simulink model "TrajectoryGenerator2DOF"  (R2023b)
settings: Solver=FixedStepDiscrete  StartTime=0.0  StopTime=1.538*1.4  FixedStep=0.002  RelTol=1e-3
undefined symbols (not defined in the file or in its folder): M_z, Smoothers, Ts
(part 1 of 3)
settings Model: Creator=simon  LastModifiedBy=simon

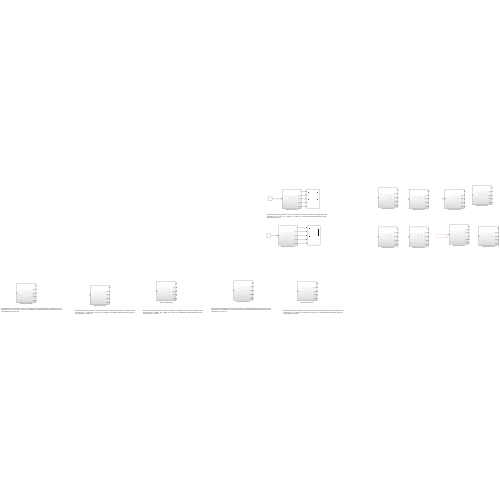
[thumbnail: Simulink's stored preview of the top-level diagram]
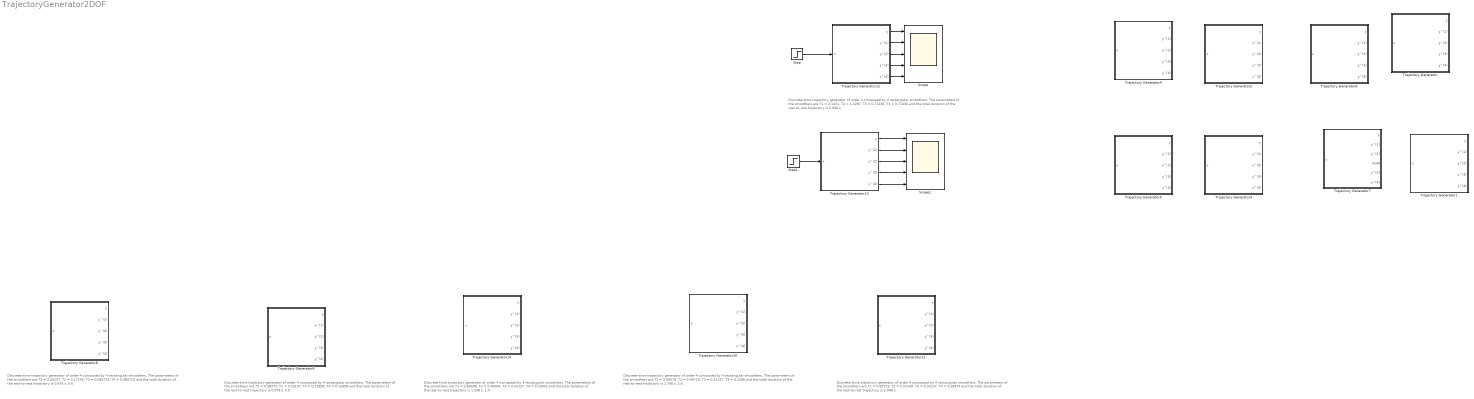
== system TrajectoryGenerator2DOF ==
  note: Discrete-time trajectory generator of order 4 composed by 4 rectangular smoothers. The parameters of the smoothers are T1 = 2.1431, T2 = 1.4287, T3 = 0.71436, T4 = 0.71436 and the total duration of the rest-to-rest trajectory is 5.006 s.
  note: Discrete-time trajectory generator of order 4 composed by 4 rectangular smoothers. The parameters of the smoothers are T1 = 0.33137, T2 = 0.17145, T3 = 0.085723, T4 = 0.085723 and the total duration of the rest-to-rest trajectory is 0.676 s. 0.6
  note: Discrete-time trajectory generator of order 4 composed by 4 rectangular smoothers. The parameters of the smoothers are T1 = 0.38575, T2 = 0.33137, T3 = 0.12858, T4 = 0.12858 and the total duration of the rest-to-rest trajectory is 0.978 s. 0.9
  note: Discrete-time trajectory generator of order 4 composed by 4 rectangular smoothers. The parameters of the smoothers are T1 = 0.68579, T2 = 0.45719, T3 = 0.33137, T4 = 0.2286 and the total duration of the rest-to-rest trajectory is 1.706 s. 1.6
  note: Discrete-time trajectory generator of order 4 composed by 4 rectangular smoothers. The parameters of the smoothers are T1 = 0.85723, T2 = 0.57149, T3 = 0.33137, T4 = 0.28574 and the total duration of the rest-to-rest trajectory is 2.048 s.
  note: Discrete-time trajectory generator of order 4 composed by 4 rectangular smoothers. The parameters of the smoothers are T1 = 0.60006, T2 = 0.40004, T3 = 0.33137, T4 = 0.20002 and the total duration of the rest-to-rest trajectory is 1.538 s. 1.4
  Scope : Scope  NumInputPorts=5
  Scope1 : Scope  NumInputPorts=5
  Step : Step  Time=0  After=0.5  SampleTime=0.002
  Step1 : Step  Time=0.4*Ts  After=-0.5  SampleTime=0.002
  Trajectory Generator : Subsystem
  Trajectory Generator1 : Subsystem
  Trajectory Generator10 : Subsystem
  Trajectory Generator11 : Subsystem
  Trajectory Generator12 : Subsystem
  Trajectory Generator13 : Subsystem
  Trajectory Generator14 : Subsystem
  Trajectory Generator2 : Subsystem
  Trajectory Generator3 : Subsystem
  Trajectory Generator4 : Subsystem
  Trajectory Generator5 : Subsystem
  Trajectory Generator6 : Subsystem
  Trajectory Generator7 : Subsystem
  Trajectory Generator8 : Subsystem
  Trajectory Generator9 : Subsystem
  wires:
  Step/1 -> Trajectory Generator12/1(x)
  Trajectory Generator12/1(y) -> Scope/1
  Trajectory Generator12/2(y^(1)) -> Scope/2
  Trajectory Generator12/3(y^(2)) -> Scope/3
  Trajectory Generator12/4(y^(3)) -> Scope/4
  Trajectory Generator12/5(y^(4)) -> Scope/5
  Step1/1 -> Trajectory Generator13/1(x)
  Trajectory Generator13/4(y^(3)) -> Scope1/4
  Trajectory Generator13/3(y^(2)) -> Scope1/3
  Trajectory Generator13/2(y^(1)) -> Scope1/2
  Trajectory Generator13/1(y) -> Scope1/1
  Trajectory Generator13/5(y^(4)) -> Scope1/5
  ? -> Trajectory Generator6/1(x)
  ? -> Trajectory Generator7/1(x)

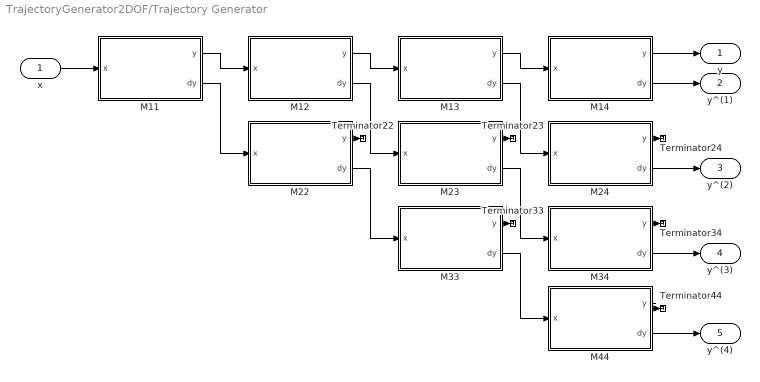
== system TrajectoryGenerator2DOF/Trajectory Generator ==
  x : Inport
  M11 : Subsystem  AncestorBlock=Smoothers/M_z  mask{N=1072, Ts=0.002, Q0=0}
      mask prompts: N "N_i"; Ts "Sampling period (Ts)"; Q0 "Initial position"
  M12 : Subsystem  AncestorBlock=Smoothers/M_z  mask{N=715, Ts=0.002, Q0=0}
      mask prompts: N "N_i"; Ts "Sampling period (Ts)"; Q0 "Initial position"
  M13 : Subsystem  AncestorBlock=Smoothers/M_z  mask{N=358, Ts=0.002, Q0=0}
      mask prompts: N "N_i"; Ts "Sampling period (Ts)"; Q0 "Initial position"
  M14 : Subsystem  AncestorBlock=Smoothers/M_z  mask{N=358, Ts=0.002, Q0=0}
      mask prompts: N "N_i"; Ts "Sampling period (Ts)"; Q0 "Initial position"
  M22 : Subsystem  AncestorBlock=Smoothers/M_z  mask{N=715, Ts=0.002, Q0=0}
      mask prompts: N "N_i"; Ts "Sampling period (Ts)"; Q0 "Initial position"
  M23 : Subsystem  AncestorBlock=Smoothers/M_z  mask{N=358, Ts=0.002, Q0=0}
      mask prompts: N "N_i"; Ts "Sampling period (Ts)"; Q0 "Initial position"
  M24 : Subsystem  AncestorBlock=Smoothers/M_z  mask{N=358, Ts=0.002, Q0=0}
      mask prompts: N "N_i"; Ts "Sampling period (Ts)"; Q0 "Initial position"
  M33 : Subsystem  AncestorBlock=Smoothers/M_z  mask{N=358, Ts=0.002, Q0=0}
      mask prompts: N "N_i"; Ts "Sampling period (Ts)"; Q0 "Initial position"
  M34 : Subsystem  AncestorBlock=Smoothers/M_z  mask{N=358, Ts=0.002, Q0=0}
      mask prompts: N "N_i"; Ts "Sampling period (Ts)"; Q0 "Initial position"
  M44 : Subsystem  AncestorBlock=Smoothers/M_z  mask{N=358, Ts=0.002, Q0=0}
      mask prompts: N "N_i"; Ts "Sampling period (Ts)"; Q0 "Initial position"
  Terminator{22..24,33..34,44} (6 alike) : Terminator
  y : Outport
  y^(1) : Outport  Port=2
  y^(2) : Outport  Port=3
  y^(3) : Outport  Port=4
  y^(4) : Outport  Port=5
  wires:
  x/1 -> M11/1(x)
  M11/1(y) -> M12/1(x)
  M12/1(y) -> M13/1(x)
  M13/1(y) -> M14/1(x)
  M11/2(dy) -> M22/1(x)
  M12/2(dy) -> M23/1(x)
  M13/2(dy) -> M24/1(x)
  M22/2(dy) -> M33/1(x)
  M23/2(dy) -> M34/1(x)
  M33/2(dy) -> M44/1(x)
  M22/1(y) -> Terminator22/1
  M23/1(y) -> Terminator23/1
  M24/1(y) -> Terminator24/1
  M33/1(y) -> Terminator33/1
  M34/1(y) -> Terminator34/1
  M44/1(y) -> Terminator44/1
  M14/1(y) -> y/1
  M14/2(dy) -> y^(1)/1
  M24/2(dy) -> y^(2)/1
  M34/2(dy) -> y^(3)/1
  M44/2(dy) -> y^(4)/1

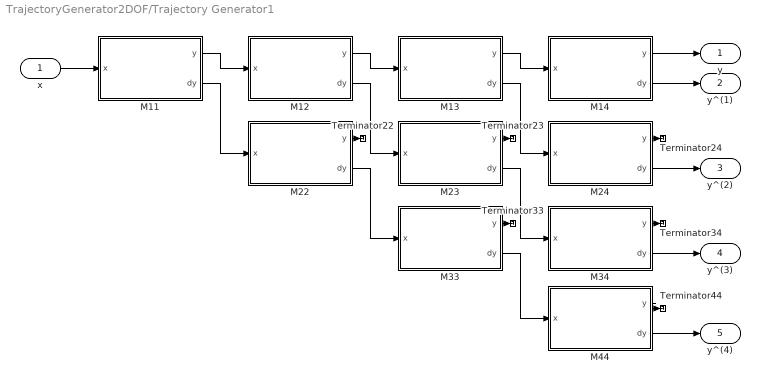
== system TrajectoryGenerator2DOF/Trajectory Generator1 ==
  x : Inport
  M11 : Subsystem  AncestorBlock=Smoothers/M_z  mask{N=1072, Ts=0.002, Q0=0}
      mask prompts: N "N_i"; Ts "Sampling period (Ts)"; Q0 "Initial position"
  M12 : Subsystem  AncestorBlock=Smoothers/M_z  mask{N=715, Ts=0.002, Q0=0}
      mask prompts: N "N_i"; Ts "Sampling period (Ts)"; Q0 "Initial position"
  M13 : Subsystem  AncestorBlock=Smoothers/M_z  mask{N=358, Ts=0.002, Q0=0}
      mask prompts: N "N_i"; Ts "Sampling period (Ts)"; Q0 "Initial position"
  M14 : Subsystem  AncestorBlock=Smoothers/M_z  mask{N=358, Ts=0.002, Q0=0}
      mask prompts: N "N_i"; Ts "Sampling period (Ts)"; Q0 "Initial position"
  M22 : Subsystem  AncestorBlock=Smoothers/M_z  mask{N=715, Ts=0.002, Q0=0}
      mask prompts: N "N_i"; Ts "Sampling period (Ts)"; Q0 "Initial position"
  M23 : Subsystem  AncestorBlock=Smoothers/M_z  mask{N=358, Ts=0.002, Q0=0}
      mask prompts: N "N_i"; Ts "Sampling period (Ts)"; Q0 "Initial position"
  M24 : Subsystem  AncestorBlock=Smoothers/M_z  mask{N=358, Ts=0.002, Q0=0}
      mask prompts: N "N_i"; Ts "Sampling period (Ts)"; Q0 "Initial position"
  M33 : Subsystem  AncestorBlock=Smoothers/M_z  mask{N=358, Ts=0.002, Q0=0}
      mask prompts: N "N_i"; Ts "Sampling period (Ts)"; Q0 "Initial position"
  M34 : Subsystem  AncestorBlock=Smoothers/M_z  mask{N=358, Ts=0.002, Q0=0}
      mask prompts: N "N_i"; Ts "Sampling period (Ts)"; Q0 "Initial position"
  M44 : Subsystem  AncestorBlock=Smoothers/M_z  mask{N=358, Ts=0.002, Q0=0}
      mask prompts: N "N_i"; Ts "Sampling period (Ts)"; Q0 "Initial position"
  Terminator{22..24,33..34,44} (6 alike) : Terminator
  y : Outport
  y^(1) : Outport  Port=2
  y^(2) : Outport  Port=3
  y^(3) : Outport  Port=4
  y^(4) : Outport  Port=5
  wires:
  M44/2(dy) -> y^(4)/1
  M34/2(dy) -> y^(3)/1
  M24/2(dy) -> y^(2)/1
  M14/2(dy) -> y^(1)/1
  M14/1(y) -> y/1
  M44/1(y) -> Terminator44/1
  M34/1(y) -> Terminator34/1
  M33/1(y) -> Terminator33/1
  M24/1(y) -> Terminator24/1
  M23/1(y) -> Terminator23/1
  M22/1(y) -> Terminator22/1
  M33/2(dy) -> M44/1(x)
  M23/2(dy) -> M34/1(x)
  M22/2(dy) -> M33/1(x)
  M13/2(dy) -> M24/1(x)
  M12/2(dy) -> M23/1(x)
  M11/2(dy) -> M22/1(x)
  M13/1(y) -> M14/1(x)
  M12/1(y) -> M13/1(x)
  M11/1(y) -> M12/1(x)
  x/1 -> M11/1(x)

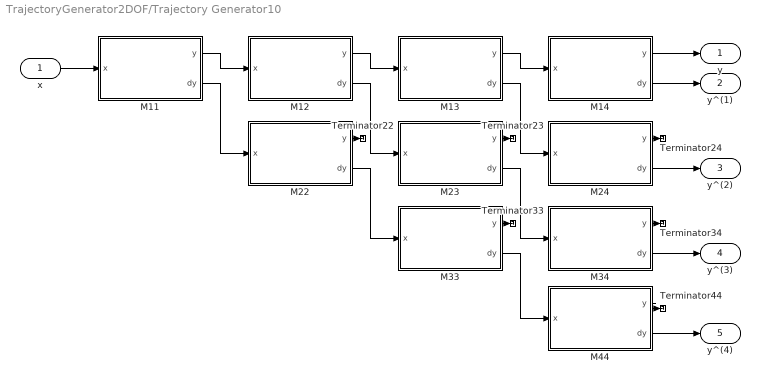
== system TrajectoryGenerator2DOF/Trajectory Generator10 ==
  x : Inport
  M11 : Subsystem  AncestorBlock=Smoothers/M_z  mask{N=343, Ts=0.002, Q0=0}
      mask prompts: N "N_i"; Ts "Sampling period (Ts)"; Q0 "Initial position"
  M12 : Subsystem  AncestorBlock=Smoothers/M_z  mask{N=229, Ts=0.002, Q0=0}
      mask prompts: N "N_i"; Ts "Sampling period (Ts)"; Q0 "Initial position"
  M13 : Subsystem  AncestorBlock=Smoothers/M_z  mask{N=166, Ts=0.002, Q0=0}
      mask prompts: N "N_i"; Ts "Sampling period (Ts)"; Q0 "Initial position"
  M14 : Subsystem  AncestorBlock=Smoothers/M_z  mask{N=115, Ts=0.002, Q0=0}
      mask prompts: N "N_i"; Ts "Sampling period (Ts)"; Q0 "Initial position"
  M22 : Subsystem  AncestorBlock=Smoothers/M_z  mask{N=229, Ts=0.002, Q0=0}
      mask prompts: N "N_i"; Ts "Sampling period (Ts)"; Q0 "Initial position"
  M23 : Subsystem  AncestorBlock=Smoothers/M_z  mask{N=166, Ts=0.002, Q0=0}
      mask prompts: N "N_i"; Ts "Sampling period (Ts)"; Q0 "Initial position"
  M24 : Subsystem  AncestorBlock=Smoothers/M_z  mask{N=115, Ts=0.002, Q0=0}
      mask prompts: N "N_i"; Ts "Sampling period (Ts)"; Q0 "Initial position"
  M33 : Subsystem  AncestorBlock=Smoothers/M_z  mask{N=166, Ts=0.002, Q0=0}
      mask prompts: N "N_i"; Ts "Sampling period (Ts)"; Q0 "Initial position"
  M34 : Subsystem  AncestorBlock=Smoothers/M_z  mask{N=115, Ts=0.002, Q0=0}
      mask prompts: N "N_i"; Ts "Sampling period (Ts)"; Q0 "Initial position"
  M44 : Subsystem  AncestorBlock=Smoothers/M_z  mask{N=115, Ts=0.002, Q0=0}
      mask prompts: N "N_i"; Ts "Sampling period (Ts)"; Q0 "Initial position"
  Terminator{22..24,33..34,44} (6 alike) : Terminator
  y : Outport
  y^(1) : Outport  Port=2
  y^(2) : Outport  Port=3
  y^(3) : Outport  Port=4
  y^(4) : Outport  Port=5
  wires:
  x/1 -> M11/1(x)
  M11/1(y) -> M12/1(x)
  M12/1(y) -> M13/1(x)
  M13/1(y) -> M14/1(x)
  M11/2(dy) -> M22/1(x)
  M12/2(dy) -> M23/1(x)
  M13/2(dy) -> M24/1(x)
  M22/2(dy) -> M33/1(x)
  M23/2(dy) -> M34/1(x)
  M33/2(dy) -> M44/1(x)
  M22/1(y) -> Terminator22/1
  M23/1(y) -> Terminator23/1
  M24/1(y) -> Terminator24/1
  M33/1(y) -> Terminator33/1
  M34/1(y) -> Terminator34/1
  M44/1(y) -> Terminator44/1
  M14/1(y) -> y/1
  M14/2(dy) -> y^(1)/1
  M24/2(dy) -> y^(2)/1
  M34/2(dy) -> y^(3)/1
  M44/2(dy) -> y^(4)/1

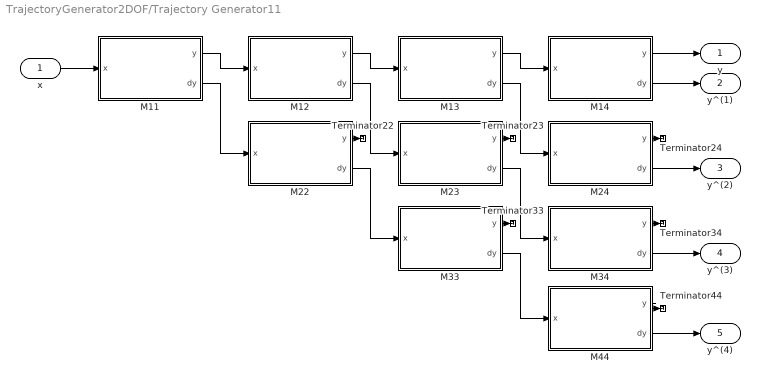
== system TrajectoryGenerator2DOF/Trajectory Generator11 ==
  x : Inport
  M11 : Subsystem  AncestorBlock=Smoothers/M_z  mask{N=429, Ts=0.002, Q0=0}
      mask prompts: N "N_i"; Ts "Sampling period (Ts)"; Q0 "Initial position"
  M12 : Subsystem  AncestorBlock=Smoothers/M_z  mask{N=286, Ts=0.002, Q0=0}
      mask prompts: N "N_i"; Ts "Sampling period (Ts)"; Q0 "Initial position"
  M13 : Subsystem  AncestorBlock=Smoothers/M_z  mask{N=166, Ts=0.002, Q0=0}
      mask prompts: N "N_i"; Ts "Sampling period (Ts)"; Q0 "Initial position"
  M14 : Subsystem  AncestorBlock=Smoothers/M_z  mask{N=143, Ts=0.002, Q0=0}
      mask prompts: N "N_i"; Ts "Sampling period (Ts)"; Q0 "Initial position"
  M22 : Subsystem  AncestorBlock=Smoothers/M_z  mask{N=286, Ts=0.002, Q0=0}
      mask prompts: N "N_i"; Ts "Sampling period (Ts)"; Q0 "Initial position"
  M23 : Subsystem  AncestorBlock=Smoothers/M_z  mask{N=166, Ts=0.002, Q0=0}
      mask prompts: N "N_i"; Ts "Sampling period (Ts)"; Q0 "Initial position"
  M24 : Subsystem  AncestorBlock=Smoothers/M_z  mask{N=143, Ts=0.002, Q0=0}
      mask prompts: N "N_i"; Ts "Sampling period (Ts)"; Q0 "Initial position"
  M33 : Subsystem  AncestorBlock=Smoothers/M_z  mask{N=166, Ts=0.002, Q0=0}
      mask prompts: N "N_i"; Ts "Sampling period (Ts)"; Q0 "Initial position"
  M34 : Subsystem  AncestorBlock=Smoothers/M_z  mask{N=143, Ts=0.002, Q0=0}
      mask prompts: N "N_i"; Ts "Sampling period (Ts)"; Q0 "Initial position"
  M44 : Subsystem  AncestorBlock=Smoothers/M_z  mask{N=143, Ts=0.002, Q0=0}
      mask prompts: N "N_i"; Ts "Sampling period (Ts)"; Q0 "Initial position"
  Terminator{22..24,33..34,44} (6 alike) : Terminator
  y : Outport
  y^(1) : Outport  Port=2
  y^(2) : Outport  Port=3
  y^(3) : Outport  Port=4
  y^(4) : Outport  Port=5
  wires:
  x/1 -> M11/1(x)
  M11/1(y) -> M12/1(x)
  M12/1(y) -> M13/1(x)
  M13/1(y) -> M14/1(x)
  M11/2(dy) -> M22/1(x)
  M12/2(dy) -> M23/1(x)
  M13/2(dy) -> M24/1(x)
  M22/2(dy) -> M33/1(x)
  M23/2(dy) -> M34/1(x)
  M33/2(dy) -> M44/1(x)
  M22/1(y) -> Terminator22/1
  M23/1(y) -> Terminator23/1
  M24/1(y) -> Terminator24/1
  M33/1(y) -> Terminator33/1
  M34/1(y) -> Terminator34/1
  M44/1(y) -> Terminator44/1
  M14/1(y) -> y/1
  M14/2(dy) -> y^(1)/1
  M24/2(dy) -> y^(2)/1
  M34/2(dy) -> y^(3)/1
  M44/2(dy) -> y^(4)/1

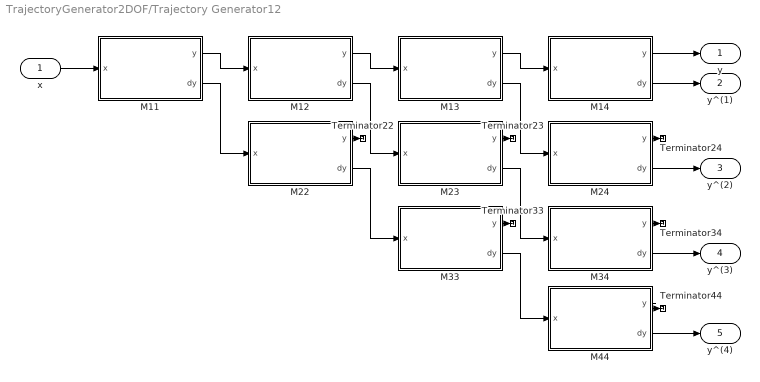
== system TrajectoryGenerator2DOF/Trajectory Generator12 ==
  x : Inport
  M11 : Subsystem  AncestorBlock=Smoothers/M_z  mask{N=301, Ts=0.002, Q0=0}
      mask prompts: N "N_i"; Ts "Sampling period (Ts)"; Q0 "Initial position"
  M12 : Subsystem  AncestorBlock=Smoothers/M_z  mask{N=201, Ts=0.002, Q0=0}
      mask prompts: N "N_i"; Ts "Sampling period (Ts)"; Q0 "Initial position"
  M13 : Subsystem  AncestorBlock=Smoothers/M_z  mask{N=166, Ts=0.002, Q0=0}
      mask prompts: N "N_i"; Ts "Sampling period (Ts)"; Q0 "Initial position"
  M14 : Subsystem  AncestorBlock=Smoothers/M_z  mask{N=101, Ts=0.002, Q0=0}
      mask prompts: N "N_i"; Ts "Sampling period (Ts)"; Q0 "Initial position"
  M22 : Subsystem  AncestorBlock=Smoothers/M_z  mask{N=201, Ts=0.002, Q0=0}
      mask prompts: N "N_i"; Ts "Sampling period (Ts)"; Q0 "Initial position"
  M23 : Subsystem  AncestorBlock=Smoothers/M_z  mask{N=166, Ts=0.002, Q0=0}
      mask prompts: N "N_i"; Ts "Sampling period (Ts)"; Q0 "Initial position"
  M24 : Subsystem  AncestorBlock=Smoothers/M_z  mask{N=101, Ts=0.002, Q0=0}
      mask prompts: N "N_i"; Ts "Sampling period (Ts)"; Q0 "Initial position"
  M33 : Subsystem  AncestorBlock=Smoothers/M_z  mask{N=166, Ts=0.002, Q0=0}
      mask prompts: N "N_i"; Ts "Sampling period (Ts)"; Q0 "Initial position"
  M34 : Subsystem  AncestorBlock=Smoothers/M_z  mask{N=101, Ts=0.002, Q0=0}
      mask prompts: N "N_i"; Ts "Sampling period (Ts)"; Q0 "Initial position"
  M44 : Subsystem  AncestorBlock=Smoothers/M_z  mask{N=101, Ts=0.002, Q0=0}
      mask prompts: N "N_i"; Ts "Sampling period (Ts)"; Q0 "Initial position"
  Terminator{22..24,33..34,44} (6 alike) : Terminator
  y : Outport
  y^(1) : Outport  Port=2
  y^(2) : Outport  Port=3
  y^(3) : Outport  Port=4
  y^(4) : Outport  Port=5
  wires:
  x/1 -> M11/1(x)
  M11/1(y) -> M12/1(x)
  M12/1(y) -> M13/1(x)
  M13/1(y) -> M14/1(x)
  M11/2(dy) -> M22/1(x)
  M12/2(dy) -> M23/1(x)
  M13/2(dy) -> M24/1(x)
  M22/2(dy) -> M33/1(x)
  M23/2(dy) -> M34/1(x)
  M33/2(dy) -> M44/1(x)
  M22/1(y) -> Terminator22/1
  M23/1(y) -> Terminator23/1
  M24/1(y) -> Terminator24/1
  M33/1(y) -> Terminator33/1
  M34/1(y) -> Terminator34/1
  M44/1(y) -> Terminator44/1
  M14/1(y) -> y/1
  M14/2(dy) -> y^(1)/1
  M24/2(dy) -> y^(2)/1
  M34/2(dy) -> y^(3)/1
  M44/2(dy) -> y^(4)/1

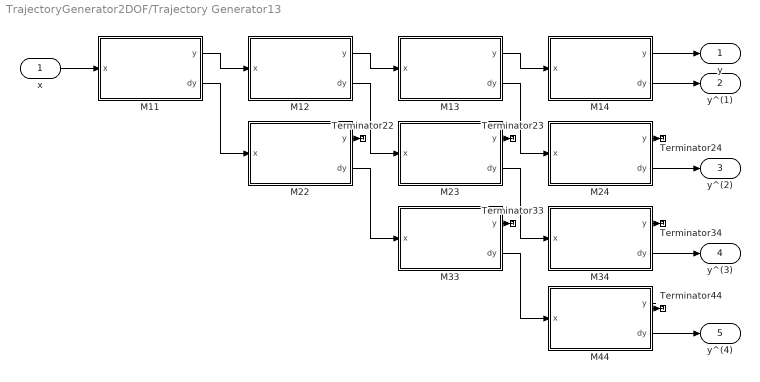
== system TrajectoryGenerator2DOF/Trajectory Generator13 ==
  x : Inport
  M11 : Subsystem  AncestorBlock=Smoothers/M_z  mask{N=301, Ts=0.002, Q0=0}
      mask prompts: N "N_i"; Ts "Sampling period (Ts)"; Q0 "Initial position"
  M12 : Subsystem  AncestorBlock=Smoothers/M_z  mask{N=201, Ts=0.002, Q0=0}
      mask prompts: N "N_i"; Ts "Sampling period (Ts)"; Q0 "Initial position"
  M13 : Subsystem  AncestorBlock=Smoothers/M_z  mask{N=166, Ts=0.002, Q0=0}
      mask prompts: N "N_i"; Ts "Sampling period (Ts)"; Q0 "Initial position"
  M14 : Subsystem  AncestorBlock=Smoothers/M_z  mask{N=101, Ts=0.002, Q0=0}
      mask prompts: N "N_i"; Ts "Sampling period (Ts)"; Q0 "Initial position"
  M22 : Subsystem  AncestorBlock=Smoothers/M_z  mask{N=201, Ts=0.002, Q0=0}
      mask prompts: N "N_i"; Ts "Sampling period (Ts)"; Q0 "Initial position"
  M23 : Subsystem  AncestorBlock=Smoothers/M_z  mask{N=166, Ts=0.002, Q0=0}
      mask prompts: N "N_i"; Ts "Sampling period (Ts)"; Q0 "Initial position"
  M24 : Subsystem  AncestorBlock=Smoothers/M_z  mask{N=101, Ts=0.002, Q0=0}
      mask prompts: N "N_i"; Ts "Sampling period (Ts)"; Q0 "Initial position"
  M33 : Subsystem  AncestorBlock=Smoothers/M_z  mask{N=166, Ts=0.002, Q0=0}
      mask prompts: N "N_i"; Ts "Sampling period (Ts)"; Q0 "Initial position"
  M34 : Subsystem  AncestorBlock=Smoothers/M_z  mask{N=101, Ts=0.002, Q0=0}
      mask prompts: N "N_i"; Ts "Sampling period (Ts)"; Q0 "Initial position"
  M44 : Subsystem  AncestorBlock=Smoothers/M_z  mask{N=101, Ts=0.002, Q0=0}
      mask prompts: N "N_i"; Ts "Sampling period (Ts)"; Q0 "Initial position"
  Terminator{22..24,33..34,44} (6 alike) : Terminator
  y : Outport
  y^(1) : Outport  Port=2
  y^(2) : Outport  Port=3
  y^(3) : Outport  Port=4
  y^(4) : Outport  Port=5
  wires:
  x/1 -> M11/1(x)
  M11/1(y) -> M12/1(x)
  M12/1(y) -> M13/1(x)
  M13/1(y) -> M14/1(x)
  M11/2(dy) -> M22/1(x)
  M12/2(dy) -> M23/1(x)
  M13/2(dy) -> M24/1(x)
  M22/2(dy) -> M33/1(x)
  M23/2(dy) -> M34/1(x)
  M33/2(dy) -> M44/1(x)
  M22/1(y) -> Terminator22/1
  M23/1(y) -> Terminator23/1
  M24/1(y) -> Terminator24/1
  M33/1(y) -> Terminator33/1
  M34/1(y) -> Terminator34/1
  M44/1(y) -> Terminator44/1
  M14/1(y) -> y/1
  M14/2(dy) -> y^(1)/1
  M24/2(dy) -> y^(2)/1
  M34/2(dy) -> y^(3)/1
  M44/2(dy) -> y^(4)/1

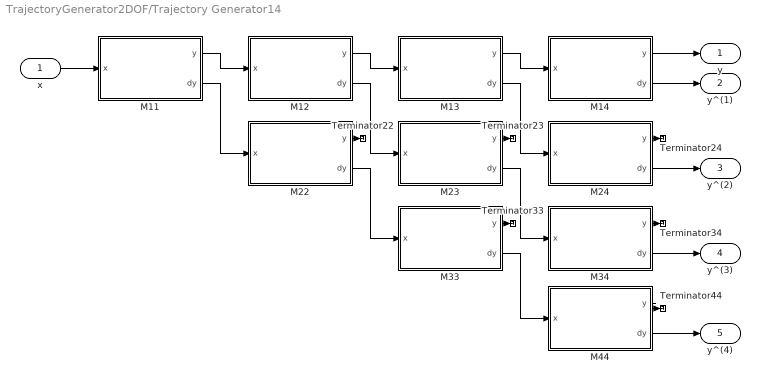
== system TrajectoryGenerator2DOF/Trajectory Generator14 ==
  x : Inport
  M11 : Subsystem  AncestorBlock=Smoothers/M_z  mask{N=301, Ts=0.002, Q0=0}
      mask prompts: N "N_i"; Ts "Sampling period (Ts)"; Q0 "Initial position"
  M12 : Subsystem  AncestorBlock=Smoothers/M_z  mask{N=201, Ts=0.002, Q0=0}
      mask prompts: N "N_i"; Ts "Sampling period (Ts)"; Q0 "Initial position"
  M13 : Subsystem  AncestorBlock=Smoothers/M_z  mask{N=166, Ts=0.002, Q0=0}
      mask prompts: N "N_i"; Ts "Sampling period (Ts)"; Q0 "Initial position"
  M14 : Subsystem  AncestorBlock=Smoothers/M_z  mask{N=101, Ts=0.002, Q0=0}
      mask prompts: N "N_i"; Ts "Sampling period (Ts)"; Q0 "Initial position"
  M22 : Subsystem  AncestorBlock=Smoothers/M_z  mask{N=201, Ts=0.002, Q0=0}
      mask prompts: N "N_i"; Ts "Sampling period (Ts)"; Q0 "Initial position"
  M23 : Subsystem  AncestorBlock=Smoothers/M_z  mask{N=166, Ts=0.002, Q0=0}
      mask prompts: N "N_i"; Ts "Sampling period (Ts)"; Q0 "Initial position"
  M24 : Subsystem  AncestorBlock=Smoothers/M_z  mask{N=101, Ts=0.002, Q0=0}
      mask prompts: N "N_i"; Ts "Sampling period (Ts)"; Q0 "Initial position"
  M33 : Subsystem  AncestorBlock=Smoothers/M_z  mask{N=166, Ts=0.002, Q0=0}
      mask prompts: N "N_i"; Ts "Sampling period (Ts)"; Q0 "Initial position"
  M34 : Subsystem  AncestorBlock=Smoothers/M_z  mask{N=101, Ts=0.002, Q0=0}
      mask prompts: N "N_i"; Ts "Sampling period (Ts)"; Q0 "Initial position"
  M44 : Subsystem  AncestorBlock=Smoothers/M_z  mask{N=101, Ts=0.002, Q0=0}
      mask prompts: N "N_i"; Ts "Sampling period (Ts)"; Q0 "Initial position"
  Terminator{22..24,33..34,44} (6 alike) : Terminator
  y : Outport
  y^(1) : Outport  Port=2
  y^(2) : Outport  Port=3
  y^(3) : Outport  Port=4
  y^(4) : Outport  Port=5
  wires:
  x/1 -> M11/1(x)
  M11/1(y) -> M12/1(x)
  M12/1(y) -> M13/1(x)
  M13/1(y) -> M14/1(x)
  M11/2(dy) -> M22/1(x)
  M12/2(dy) -> M23/1(x)
  M13/2(dy) -> M24/1(x)
  M22/2(dy) -> M33/1(x)
  M23/2(dy) -> M34/1(x)
  M33/2(dy) -> M44/1(x)
  M22/1(y) -> Terminator22/1
  M23/1(y) -> Terminator23/1
  M24/1(y) -> Terminator24/1
  M33/1(y) -> Terminator33/1
  M34/1(y) -> Terminator34/1
  M44/1(y) -> Terminator44/1
  M14/1(y) -> y/1
  M14/2(dy) -> y^(1)/1
  M24/2(dy) -> y^(2)/1
  M34/2(dy) -> y^(3)/1
  M44/2(dy) -> y^(4)/1

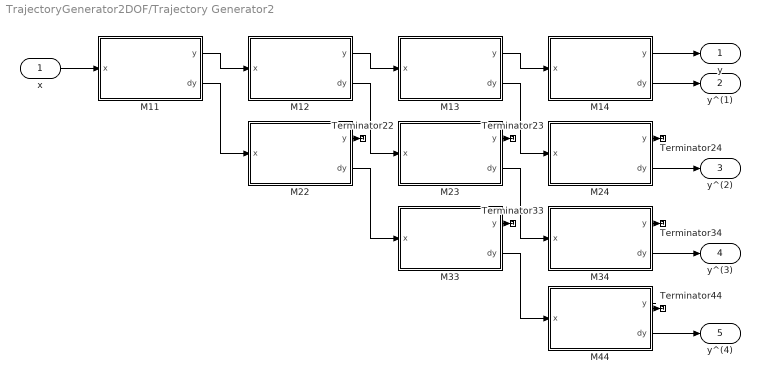
== system TrajectoryGenerator2DOF/Trajectory Generator2 ==
  x : Inport
  M11 : Subsystem  AncestorBlock=Smoothers/M_z  mask{N=215, Ts=0.002, Q0=0}
      mask prompts: N "N_i"; Ts "Sampling period (Ts)"; Q0 "Initial position"
  M12 : Subsystem  AncestorBlock=Smoothers/M_z  mask{N=143, Ts=0.002, Q0=0}
      mask prompts: N "N_i"; Ts "Sampling period (Ts)"; Q0 "Initial position"
  M13 : Subsystem  AncestorBlock=Smoothers/M_z  mask{N=72, Ts=0.002, Q0=0}
      mask prompts: N "N_i"; Ts "Sampling period (Ts)"; Q0 "Initial position"
  M14 : Subsystem  AncestorBlock=Smoothers/M_z  mask{N=72, Ts=0.002, Q0=0}
      mask prompts: N "N_i"; Ts "Sampling period (Ts)"; Q0 "Initial position"
  M22 : Subsystem  AncestorBlock=Smoothers/M_z  mask{N=143, Ts=0.002, Q0=0}
      mask prompts: N "N_i"; Ts "Sampling period (Ts)"; Q0 "Initial position"
  M23 : Subsystem  AncestorBlock=Smoothers/M_z  mask{N=72, Ts=0.002, Q0=0}
      mask prompts: N "N_i"; Ts "Sampling period (Ts)"; Q0 "Initial position"
  M24 : Subsystem  AncestorBlock=Smoothers/M_z  mask{N=72, Ts=0.002, Q0=0}
      mask prompts: N "N_i"; Ts "Sampling period (Ts)"; Q0 "Initial position"
  M33 : Subsystem  AncestorBlock=Smoothers/M_z  mask{N=72, Ts=0.002, Q0=0}
      mask prompts: N "N_i"; Ts "Sampling period (Ts)"; Q0 "Initial position"
  M34 : Subsystem  AncestorBlock=Smoothers/M_z  mask{N=72, Ts=0.002, Q0=0}
      mask prompts: N "N_i"; Ts "Sampling period (Ts)"; Q0 "Initial position"
  M44 : Subsystem  AncestorBlock=Smoothers/M_z  mask{N=72, Ts=0.002, Q0=0}
      mask prompts: N "N_i"; Ts "Sampling period (Ts)"; Q0 "Initial position"
  Terminator{22..24,33..34,44} (6 alike) : Terminator
  y : Outport
  y^(1) : Outport  Port=2
  y^(2) : Outport  Port=3
  y^(3) : Outport  Port=4
  y^(4) : Outport  Port=5
  wires:
  x/1 -> M11/1(x)
  M11/1(y) -> M12/1(x)
  M12/1(y) -> M13/1(x)
  M13/1(y) -> M14/1(x)
  M11/2(dy) -> M22/1(x)
  M12/2(dy) -> M23/1(x)
  M13/2(dy) -> M24/1(x)
  M22/2(dy) -> M33/1(x)
  M23/2(dy) -> M34/1(x)
  M33/2(dy) -> M44/1(x)
  M22/1(y) -> Terminator22/1
  M23/1(y) -> Terminator23/1
  M24/1(y) -> Terminator24/1
  M33/1(y) -> Terminator33/1
  M34/1(y) -> Terminator34/1
  M44/1(y) -> Terminator44/1
  M14/1(y) -> y/1
  M14/2(dy) -> y^(1)/1
  M24/2(dy) -> y^(2)/1
  M34/2(dy) -> y^(3)/1
  M44/2(dy) -> y^(4)/1

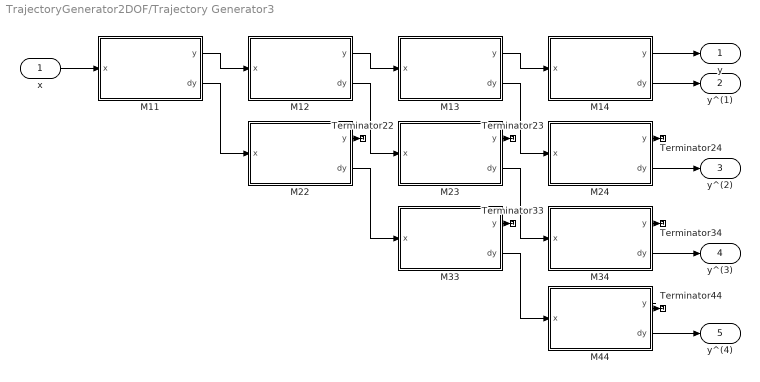
== system TrajectoryGenerator2DOF/Trajectory Generator3 ==
  x : Inport
  M11 : Subsystem  AncestorBlock=Smoothers/M_z  mask{N=215, Ts=0.002, Q0=0}
      mask prompts: N "N_i"; Ts "Sampling period (Ts)"; Q0 "Initial position"
  M12 : Subsystem  AncestorBlock=Smoothers/M_z  mask{N=143, Ts=0.002, Q0=0}
      mask prompts: N "N_i"; Ts "Sampling period (Ts)"; Q0 "Initial position"
  M13 : Subsystem  AncestorBlock=Smoothers/M_z  mask{N=72, Ts=0.002, Q0=0}
      mask prompts: N "N_i"; Ts "Sampling period (Ts)"; Q0 "Initial position"
  M14 : Subsystem  AncestorBlock=Smoothers/M_z  mask{N=72, Ts=0.002, Q0=0}
      mask prompts: N "N_i"; Ts "Sampling period (Ts)"; Q0 "Initial position"
  M22 : Subsystem  AncestorBlock=Smoothers/M_z  mask{N=143, Ts=0.002, Q0=0}
      mask prompts: N "N_i"; Ts "Sampling period (Ts)"; Q0 "Initial position"
  M23 : Subsystem  AncestorBlock=Smoothers/M_z  mask{N=72, Ts=0.002, Q0=0}
      mask prompts: N "N_i"; Ts "Sampling period (Ts)"; Q0 "Initial position"
  M24 : Subsystem  AncestorBlock=Smoothers/M_z  mask{N=72, Ts=0.002, Q0=0}
      mask prompts: N "N_i"; Ts "Sampling period (Ts)"; Q0 "Initial position"
  M33 : Subsystem  AncestorBlock=Smoothers/M_z  mask{N=72, Ts=0.002, Q0=0}
      mask prompts: N "N_i"; Ts "Sampling period (Ts)"; Q0 "Initial position"
  M34 : Subsystem  AncestorBlock=Smoothers/M_z  mask{N=72, Ts=0.002, Q0=0}
      mask prompts: N "N_i"; Ts "Sampling period (Ts)"; Q0 "Initial position"
  M44 : Subsystem  AncestorBlock=Smoothers/M_z  mask{N=72, Ts=0.002, Q0=0}
      mask prompts: N "N_i"; Ts "Sampling period (Ts)"; Q0 "Initial position"
  Terminator{22..24,33..34,44} (6 alike) : Terminator
  y : Outport
  y^(1) : Outport  Port=2
  y^(2) : Outport  Port=3
  y^(3) : Outport  Port=4
  y^(4) : Outport  Port=5
  wires:
  x/1 -> M11/1(x)
  M11/1(y) -> M12/1(x)
  M12/1(y) -> M13/1(x)
  M13/1(y) -> M14/1(x)
  M11/2(dy) -> M22/1(x)
  M12/2(dy) -> M23/1(x)
  M13/2(dy) -> M24/1(x)
  M22/2(dy) -> M33/1(x)
  M23/2(dy) -> M34/1(x)
  M33/2(dy) -> M44/1(x)
  M22/1(y) -> Terminator22/1
  M23/1(y) -> Terminator23/1
  M24/1(y) -> Terminator24/1
  M33/1(y) -> Terminator33/1
  M34/1(y) -> Terminator34/1
  M44/1(y) -> Terminator44/1
  M14/1(y) -> y/1
  M14/2(dy) -> y^(1)/1
  M24/2(dy) -> y^(2)/1
  M34/2(dy) -> y^(3)/1
  M44/2(dy) -> y^(4)/1

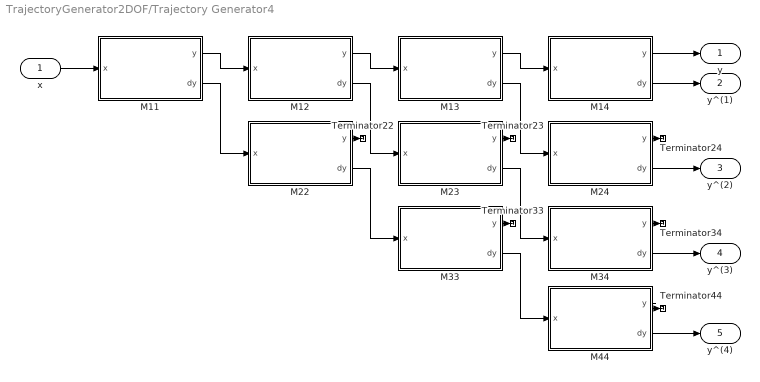
== system TrajectoryGenerator2DOF/Trajectory Generator4 ==
  x : Inport
  M11 : Subsystem  AncestorBlock=Smoothers/M_z  mask{N=429, Ts=0.002, Q0=0}
      mask prompts: N "N_i"; Ts "Sampling period (Ts)"; Q0 "Initial position"
  M12 : Subsystem  AncestorBlock=Smoothers/M_z  mask{N=286, Ts=0.002, Q0=0}
      mask prompts: N "N_i"; Ts "Sampling period (Ts)"; Q0 "Initial position"
  M13 : Subsystem  AncestorBlock=Smoothers/M_z  mask{N=143, Ts=0.002, Q0=0}
      mask prompts: N "N_i"; Ts "Sampling period (Ts)"; Q0 "Initial position"
  M14 : Subsystem  AncestorBlock=Smoothers/M_z  mask{N=143, Ts=0.002, Q0=0}
      mask prompts: N "N_i"; Ts "Sampling period (Ts)"; Q0 "Initial position"
  M22 : Subsystem  AncestorBlock=Smoothers/M_z  mask{N=286, Ts=0.002, Q0=0}
      mask prompts: N "N_i"; Ts "Sampling period (Ts)"; Q0 "Initial position"
  M23 : Subsystem  AncestorBlock=Smoothers/M_z  mask{N=143, Ts=0.002, Q0=0}
      mask prompts: N "N_i"; Ts "Sampling period (Ts)"; Q0 "Initial position"
  M24 : Subsystem  AncestorBlock=Smoothers/M_z  mask{N=143, Ts=0.002, Q0=0}
      mask prompts: N "N_i"; Ts "Sampling period (Ts)"; Q0 "Initial position"
  M33 : Subsystem  AncestorBlock=Smoothers/M_z  mask{N=143, Ts=0.002, Q0=0}
      mask prompts: N "N_i"; Ts "Sampling period (Ts)"; Q0 "Initial position"
  M34 : Subsystem  AncestorBlock=Smoothers/M_z  mask{N=143, Ts=0.002, Q0=0}
      mask prompts: N "N_i"; Ts "Sampling period (Ts)"; Q0 "Initial position"
  M44 : Subsystem  AncestorBlock=Smoothers/M_z  mask{N=143, Ts=0.002, Q0=0}
      mask prompts: N "N_i"; Ts "Sampling period (Ts)"; Q0 "Initial position"
  Terminator{22..24,33..34,44} (6 alike) : Terminator
  y : Outport
  y^(1) : Outport  Port=2
  y^(2) : Outport  Port=3
  y^(3) : Outport  Port=4
  y^(4) : Outport  Port=5
  wires:
  x/1 -> M11/1(x)
  M11/1(y) -> M12/1(x)
  M12/1(y) -> M13/1(x)
  M13/1(y) -> M14/1(x)
  M11/2(dy) -> M22/1(x)
  M12/2(dy) -> M23/1(x)
  M13/2(dy) -> M24/1(x)
  M22/2(dy) -> M33/1(x)
  M23/2(dy) -> M34/1(x)
  M33/2(dy) -> M44/1(x)
  M22/1(y) -> Terminator22/1
  M23/1(y) -> Terminator23/1
  M24/1(y) -> Terminator24/1
  M33/1(y) -> Terminator33/1
  M34/1(y) -> Terminator34/1
  M44/1(y) -> Terminator44/1
  M14/1(y) -> y/1
  M14/2(dy) -> y^(1)/1
  M24/2(dy) -> y^(2)/1
  M34/2(dy) -> y^(3)/1
  M44/2(dy) -> y^(4)/1

== system TrajectoryGenerator2DOF/Trajectory Generator5 ==
  x : Inport
  M11 : Subsystem  AncestorBlock=Smoothers/M_z  mask{N=429, Ts=0.002, Q0=0}
      mask prompts: N "N_i"; Ts "Sampling period (Ts)"; Q0 "Initial position"
  M12 : Subsystem  AncestorBlock=Smoothers/M_z  mask{N=286, Ts=0.002, Q0=0}
      mask prompts: N "N_i"; Ts "Sampling period (Ts)"; Q0 "Initial position"
  M13 : Subsystem  AncestorBlock=Smoothers/M_z  mask{N=143, Ts=0.002, Q0=0}
      mask prompts: N "N_i"; Ts "Sampling period (Ts)"; Q0 "Initial position"
  M14 : Subsystem  AncestorBlock=Smoothers/M_z  mask{N=143, Ts=0.002, Q0=0}
      mask prompts: N "N_i"; Ts "Sampling period (Ts)"; Q0 "Initial position"
  M22 : Subsystem  AncestorBlock=Smoothers/M_z  mask{N=286, Ts=0.002, Q0=0}
      mask prompts: N "N_i"; Ts "Sampling period (Ts)"; Q0 "Initial position"
  M23 : Subsystem  AncestorBlock=Smoothers/M_z  mask{N=143, Ts=0.002, Q0=0}
      mask prompts: N "N_i"; Ts "Sampling period (Ts)"; Q0 "Initial position"
  M24 : Subsystem  AncestorBlock=Smoothers/M_z  mask{N=143, Ts=0.002, Q0=0}
      mask prompts: N "N_i"; Ts "Sampling period (Ts)"; Q0 "Initial position"
  M33 : Subsystem  AncestorBlock=Smoothers/M_z  mask{N=143, Ts=0.002, Q0=0}
      mask prompts: N "N_i"; Ts "Sampling period (Ts)"; Q0 "Initial position"
  M34 : Subsystem  AncestorBlock=Smoothers/M_z  mask{N=143, Ts=0.002, Q0=0}
      mask prompts: N "N_i"; Ts "Sampling period (Ts)"; Q0 "Initial position"
  M44 : Subsystem  AncestorBlock=Smoothers/M_z  mask{N=143, Ts=0.002, Q0=0}
      mask prompts: N "N_i"; Ts "Sampling period (Ts)"; Q0 "Initial position"
  Terminator{22..24,33..34,44} (6 alike) : Terminator
  y : Outport
  y^(1) : Outport  Port=2
  y^(2) : Outport  Port=3
  y^(3) : Outport  Port=4
  y^(4) : Outport  Port=5
  wires:
  x/1 -> M11/1(x)
  M11/1(y) -> M12/1(x)
  M12/1(y) -> M13/1(x)
  M13/1(y) -> M14/1(x)
  M11/2(dy) -> M22/1(x)
  M12/2(dy) -> M23/1(x)
  M13/2(dy) -> M24/1(x)
  M22/2(dy) -> M33/1(x)
  M23/2(dy) -> M34/1(x)
  M33/2(dy) -> M44/1(x)
  M22/1(y) -> Terminator22/1
  M23/1(y) -> Terminator23/1
  M24/1(y) -> Terminator24/1
  M33/1(y) -> Terminator33/1
  M34/1(y) -> Terminator34/1
  M44/1(y) -> Terminator44/1
  M14/1(y) -> y/1
  M14/2(dy) -> y^(1)/1
  M24/2(dy) -> y^(2)/1
  M34/2(dy) -> y^(3)/1
  M44/2(dy) -> y^(4)/1

== system TrajectoryGenerator2DOF/Trajectory Generator6 ==
  x : Inport
  M11 : Subsystem  AncestorBlock=Smoothers/M_z  mask{N=643, Ts=0.002, Q0=0}
      mask prompts: N "N_i"; Ts "Sampling period (Ts)"; Q0 "Initial position"
  M12 : Subsystem  AncestorBlock=Smoothers/M_z  mask{N=429, Ts=0.002, Q0=0}
      mask prompts: N "N_i"; Ts "Sampling period (Ts)"; Q0 "Initial position"
  M13 : Subsystem  AncestorBlock=Smoothers/M_z  mask{N=215, Ts=0.002, Q0=0}
      mask prompts: N "N_i"; Ts "Sampling period (Ts)"; Q0 "Initial position"
  M14 : Subsystem  AncestorBlock=Smoothers/M_z  mask{N=215, Ts=0.002, Q0=0}
      mask prompts: N "N_i"; Ts "Sampling period (Ts)"; Q0 "Initial position"
  M22 : Subsystem  AncestorBlock=Smoothers/M_z  mask{N=429, Ts=0.002, Q0=0}
      mask prompts: N "N_i"; Ts "Sampling period (Ts)"; Q0 "Initial position"
  M23 : Subsystem  AncestorBlock=Smoothers/M_z  mask{N=215, Ts=0.002, Q0=0}
      mask prompts: N "N_i"; Ts "Sampling period (Ts)"; Q0 "Initial position"
  M24 : Subsystem  AncestorBlock=Smoothers/M_z  mask{N=215, Ts=0.002, Q0=0}
      mask prompts: N "N_i"; Ts "Sampling period (Ts)"; Q0 "Initial position"
  M33 : Subsystem  AncestorBlock=Smoothers/M_z  mask{N=215, Ts=0.002, Q0=0}
      mask prompts: N "N_i"; Ts "Sampling period (Ts)"; Q0 "Initial position"
  M34 : Subsystem  AncestorBlock=Smoothers/M_z  mask{N=215, Ts=0.002, Q0=0}
      mask prompts: N "N_i"; Ts "Sampling period (Ts)"; Q0 "Initial position"
  M44 : Subsystem  AncestorBlock=Smoothers/M_z  mask{N=215, Ts=0.002, Q0=0}
      mask prompts: N "N_i"; Ts "Sampling period (Ts)"; Q0 "Initial position"
  Terminator{22..24,33..34,44} (6 alike) : Terminator
  y : Outport
  y^(1) : Outport  Port=2
  y^(2) : Outport  Port=3
  y^(3) : Outport  Port=4
  y^(4) : Outport  Port=5
  wires:
  x/1 -> M11/1(x)
  M11/1(y) -> M12/1(x)
  M12/1(y) -> M13/1(x)
  M13/1(y) -> M14/1(x)
  M11/2(dy) -> M22/1(x)
  M12/2(dy) -> M23/1(x)
  M13/2(dy) -> M24/1(x)
  M22/2(dy) -> M33/1(x)
  M23/2(dy) -> M34/1(x)
  M33/2(dy) -> M44/1(x)
  M22/1(y) -> Terminator22/1
  M23/1(y) -> Terminator23/1
  M24/1(y) -> Terminator24/1
  M33/1(y) -> Terminator33/1
  M34/1(y) -> Terminator34/1
  M44/1(y) -> Terminator44/1
  M14/1(y) -> y/1
  M14/2(dy) -> y^(1)/1
  M24/2(dy) -> y^(2)/1
  M34/2(dy) -> y^(3)/1
  M44/2(dy) -> y^(4)/1

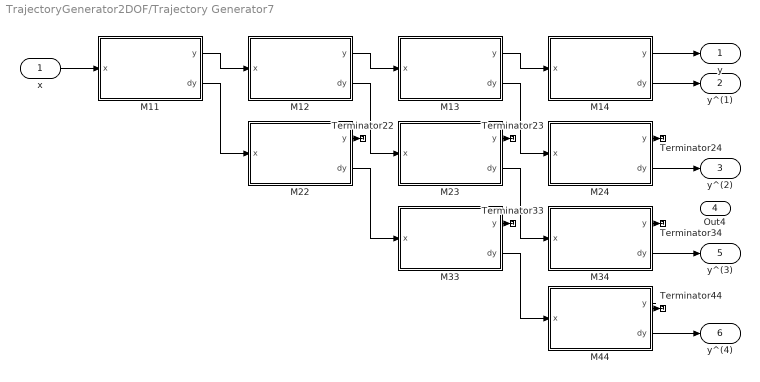
== system TrajectoryGenerator2DOF/Trajectory Generator7 ==
  x : Inport
  M11 : Subsystem  AncestorBlock=Smoothers/M_z  mask{N=643, Ts=0.002, Q0=0}
      mask prompts: N "N_i"; Ts "Sampling period (Ts)"; Q0 "Initial position"
  M12 : Subsystem  AncestorBlock=Smoothers/M_z  mask{N=429, Ts=0.002, Q0=0}
      mask prompts: N "N_i"; Ts "Sampling period (Ts)"; Q0 "Initial position"
  M13 : Subsystem  AncestorBlock=Smoothers/M_z  mask{N=215, Ts=0.002, Q0=0}
      mask prompts: N "N_i"; Ts "Sampling period (Ts)"; Q0 "Initial position"
  M14 : Subsystem  AncestorBlock=Smoothers/M_z  mask{N=215, Ts=0.002, Q0=0}
      mask prompts: N "N_i"; Ts "Sampling period (Ts)"; Q0 "Initial position"
  M22 : Subsystem  AncestorBlock=Smoothers/M_z  mask{N=429, Ts=0.002, Q0=0}
      mask prompts: N "N_i"; Ts "Sampling period (Ts)"; Q0 "Initial position"
  M23 : Subsystem  AncestorBlock=Smoothers/M_z  mask{N=215, Ts=0.002, Q0=0}
      mask prompts: N "N_i"; Ts "Sampling period (Ts)"; Q0 "Initial position"
  M24 : Subsystem  AncestorBlock=Smoothers/M_z  mask{N=215, Ts=0.002, Q0=0}
      mask prompts: N "N_i"; Ts "Sampling period (Ts)"; Q0 "Initial position"
  M33 : Subsystem  AncestorBlock=Smoothers/M_z  mask{N=215, Ts=0.002, Q0=0}
      mask prompts: N "N_i"; Ts "Sampling period (Ts)"; Q0 "Initial position"
  M34 : Subsystem  AncestorBlock=Smoothers/M_z  mask{N=215, Ts=0.002, Q0=0}
      mask prompts: N "N_i"; Ts "Sampling period (Ts)"; Q0 "Initial position"
  M44 : Subsystem  AncestorBlock=Smoothers/M_z  mask{N=215, Ts=0.002, Q0=0}
      mask prompts: N "N_i"; Ts "Sampling period (Ts)"; Q0 "Initial position"
  Terminator{22..24,33..34,44} (6 alike) : Terminator
  y : Outport
  y^(1) : Outport  Port=2
  y^(2) : Outport  Port=3
  Out4 : Outport  Port=4
  y^(3) : Outport  Port=5
  y^(4) : Outport  Port=6
  wires:
  x/1 -> M11/1(x)
  M11/1(y) -> M12/1(x)
  M12/1(y) -> M13/1(x)
  M13/1(y) -> M14/1(x)
  M11/2(dy) -> M22/1(x)
  M12/2(dy) -> M23/1(x)
  M13/2(dy) -> M24/1(x)
  M22/2(dy) -> M33/1(x)
  M23/2(dy) -> M34/1(x)
  M33/2(dy) -> M44/1(x)
  M22/1(y) -> Terminator22/1
  M23/1(y) -> Terminator23/1
  M24/1(y) -> Terminator24/1
  M33/1(y) -> Terminator33/1
  M34/1(y) -> Terminator34/1
  M44/1(y) -> Terminator44/1
  M14/1(y) -> y/1
  M14/2(dy) -> y^(1)/1
  M24/2(dy) -> y^(2)/1
  M34/2(dy) -> y^(3)/1
  M44/2(dy) -> y^(4)/1

== system TrajectoryGenerator2DOF/Trajectory Generator8 ==
  x : Inport
  M11 : Subsystem  AncestorBlock=Smoothers/M_z  mask{N=166, Ts=0.002, Q0=0}
      mask prompts: N "N_i"; Ts "Sampling period (Ts)"; Q0 "Initial position"
  M12 : Subsystem  AncestorBlock=Smoothers/M_z  mask{N=86, Ts=0.002, Q0=0}
      mask prompts: N "N_i"; Ts "Sampling period (Ts)"; Q0 "Initial position"
  M13 : Subsystem  AncestorBlock=Smoothers/M_z  mask{N=43, Ts=0.002, Q0=0}
      mask prompts: N "N_i"; Ts "Sampling period (Ts)"; Q0 "Initial position"
  M14 : Subsystem  AncestorBlock=Smoothers/M_z  mask{N=43, Ts=0.002, Q0=0}
      mask prompts: N "N_i"; Ts "Sampling period (Ts)"; Q0 "Initial position"
  M22 : Subsystem  AncestorBlock=Smoothers/M_z  mask{N=86, Ts=0.002, Q0=0}
      mask prompts: N "N_i"; Ts "Sampling period (Ts)"; Q0 "Initial position"
  M23 : Subsystem  AncestorBlock=Smoothers/M_z  mask{N=43, Ts=0.002, Q0=0}
      mask prompts: N "N_i"; Ts "Sampling period (Ts)"; Q0 "Initial position"
  M24 : Subsystem  AncestorBlock=Smoothers/M_z  mask{N=43, Ts=0.002, Q0=0}
      mask prompts: N "N_i"; Ts "Sampling period (Ts)"; Q0 "Initial position"
  M33 : Subsystem  AncestorBlock=Smoothers/M_z  mask{N=43, Ts=0.002, Q0=0}
      mask prompts: N "N_i"; Ts "Sampling period (Ts)"; Q0 "Initial position"
  M34 : Subsystem  AncestorBlock=Smoothers/M_z  mask{N=43, Ts=0.002, Q0=0}
      mask prompts: N "N_i"; Ts "Sampling period (Ts)"; Q0 "Initial position"
  M44 : Subsystem  AncestorBlock=Smoothers/M_z  mask{N=43, Ts=0.002, Q0=0}
      mask prompts: N "N_i"; Ts "Sampling period (Ts)"; Q0 "Initial position"
  Terminator{22..24,33..34,44} (6 alike) : Terminator
  y : Outport
  y^(1) : Outport  Port=2
  y^(2) : Outport  Port=3
  y^(3) : Outport  Port=4
  y^(4) : Outport  Port=5
  wires:
  x/1 -> M11/1(x)
  M11/1(y) -> M12/1(x)
  M12/1(y) -> M13/1(x)
  M13/1(y) -> M14/1(x)
  M11/2(dy) -> M22/1(x)
  M12/2(dy) -> M23/1(x)
  M13/2(dy) -> M24/1(x)
  M22/2(dy) -> M33/1(x)
  M23/2(dy) -> M34/1(x)
  M33/2(dy) -> M44/1(x)
  M22/1(y) -> Terminator22/1
  M23/1(y) -> Terminator23/1
  M24/1(y) -> Terminator24/1
  M33/1(y) -> Terminator33/1
  M34/1(y) -> Terminator34/1
  M44/1(y) -> Terminator44/1
  M14/1(y) -> y/1
  M14/2(dy) -> y^(1)/1
  M24/2(dy) -> y^(2)/1
  M34/2(dy) -> y^(3)/1
  M44/2(dy) -> y^(4)/1

== system TrajectoryGenerator2DOF/Trajectory Generator9 ==
  x : Inport
  M11 : Subsystem  AncestorBlock=Smoothers/M_z  mask{N=193, Ts=0.002, Q0=0}
      mask prompts: N "N_i"; Ts "Sampling period (Ts)"; Q0 "Initial position"
  M12 : Subsystem  AncestorBlock=Smoothers/M_z  mask{N=166, Ts=0.002, Q0=0}
      mask prompts: N "N_i"; Ts "Sampling period (Ts)"; Q0 "Initial position"
  M13 : Subsystem  AncestorBlock=Smoothers/M_z  mask{N=65, Ts=0.002, Q0=0}
      mask prompts: N "N_i"; Ts "Sampling period (Ts)"; Q0 "Initial position"
  M14 : Subsystem  AncestorBlock=Smoothers/M_z  mask{N=65, Ts=0.002, Q0=0}
      mask prompts: N "N_i"; Ts "Sampling period (Ts)"; Q0 "Initial position"
  M22 : Subsystem  AncestorBlock=Smoothers/M_z  mask{N=166, Ts=0.002, Q0=0}
      mask prompts: N "N_i"; Ts "Sampling period (Ts)"; Q0 "Initial position"
  M23 : Subsystem  AncestorBlock=Smoothers/M_z  mask{N=65, Ts=0.002, Q0=0}
      mask prompts: N "N_i"; Ts "Sampling period (Ts)"; Q0 "Initial position"
  M24 : Subsystem  AncestorBlock=Smoothers/M_z  mask{N=65, Ts=0.002, Q0=0}
      mask prompts: N "N_i"; Ts "Sampling period (Ts)"; Q0 "Initial position"
  M33 : Subsystem  AncestorBlock=Smoothers/M_z  mask{N=65, Ts=0.002, Q0=0}
      mask prompts: N "N_i"; Ts "Sampling period (Ts)"; Q0 "Initial position"
  M34 : Subsystem  AncestorBlock=Smoothers/M_z  mask{N=65, Ts=0.002, Q0=0}
      mask prompts: N "N_i"; Ts "Sampling period (Ts)"; Q0 "Initial position"
  M44 : Subsystem  AncestorBlock=Smoothers/M_z  mask{N=65, Ts=0.002, Q0=0}
      mask prompts: N "N_i"; Ts "Sampling period (Ts)"; Q0 "Initial position"
  Terminator{22..24,33..34,44} (6 alike) : Terminator
  y : Outport
  y^(1) : Outport  Port=2
  y^(2) : Outport  Port=3
  y^(3) : Outport  Port=4
  y^(4) : Outport  Port=5
  wires:
  x/1 -> M11/1(x)
  M11/1(y) -> M12/1(x)
  M12/1(y) -> M13/1(x)
  M13/1(y) -> M14/1(x)
  M11/2(dy) -> M22/1(x)
  M12/2(dy) -> M23/1(x)
  M13/2(dy) -> M24/1(x)
  M22/2(dy) -> M33/1(x)
  M23/2(dy) -> M34/1(x)
  M33/2(dy) -> M44/1(x)
  M22/1(y) -> Terminator22/1
  M23/1(y) -> Terminator23/1
  M24/1(y) -> Terminator24/1
  M33/1(y) -> Terminator33/1
  M34/1(y) -> Terminator34/1
  M44/1(y) -> Terminator44/1
  M14/1(y) -> y/1
  M14/2(dy) -> y^(1)/1
  M24/2(dy) -> y^(2)/1
  M34/2(dy) -> y^(3)/1
  M44/2(dy) -> y^(4)/1

== system TrajectoryGenerator2DOF/Trajectory Generator/M11 ==
  x : Inport
  Discrete FIR Filter1 : DiscreteFir  Coefficients=1/N/Ts*[1 zeros(1,N-1) -1]  InitialStates=Q0  SampleTime=Ts
  Discrete Filter : DiscreteFilter  Numerator=[0 Ts]  Denominator=[1 -1]  InitialStates=Q0  SampleTime=Ts
  y : Outport
  dy : Outport  Port=2
  wires:
  Discrete FIR Filter1/1 -> Discrete Filter/1, dy/1
  x/1 -> Discrete FIR Filter1/1
  Discrete Filter/1 -> y/1

== system TrajectoryGenerator2DOF/Trajectory Generator/M12 ==
  x : Inport
  Discrete FIR Filter1 : DiscreteFir  Coefficients=1/N/Ts*[1 zeros(1,N-1) -1]  InitialStates=Q0  SampleTime=Ts
  Discrete Filter : DiscreteFilter  Numerator=[0 Ts]  Denominator=[1 -1]  InitialStates=Q0  SampleTime=Ts
  y : Outport
  dy : Outport  Port=2
  wires:
  Discrete FIR Filter1/1 -> Discrete Filter/1, dy/1
  x/1 -> Discrete FIR Filter1/1
  Discrete Filter/1 -> y/1

== system TrajectoryGenerator2DOF/Trajectory Generator/M13 ==
  x : Inport
  Discrete FIR Filter1 : DiscreteFir  Coefficients=1/N/Ts*[1 zeros(1,N-1) -1]  InitialStates=Q0  SampleTime=Ts
  Discrete Filter : DiscreteFilter  Numerator=[0 Ts]  Denominator=[1 -1]  InitialStates=Q0  SampleTime=Ts
  y : Outport
  dy : Outport  Port=2
  wires:
  Discrete FIR Filter1/1 -> Discrete Filter/1, dy/1
  x/1 -> Discrete FIR Filter1/1
  Discrete Filter/1 -> y/1

== system TrajectoryGenerator2DOF/Trajectory Generator/M14 ==
  x : Inport
  Discrete FIR Filter1 : DiscreteFir  Coefficients=1/N/Ts*[1 zeros(1,N-1) -1]  InitialStates=Q0  SampleTime=Ts
  Discrete Filter : DiscreteFilter  Numerator=[0 Ts]  Denominator=[1 -1]  InitialStates=Q0  SampleTime=Ts
  y : Outport
  dy : Outport  Port=2
  wires:
  Discrete FIR Filter1/1 -> Discrete Filter/1, dy/1
  x/1 -> Discrete FIR Filter1/1
  Discrete Filter/1 -> y/1

== system TrajectoryGenerator2DOF/Trajectory Generator/M22 ==
  x : Inport
  Discrete FIR Filter1 : DiscreteFir  Coefficients=1/N/Ts*[1 zeros(1,N-1) -1]  InitialStates=Q0  SampleTime=Ts
  Discrete Filter : DiscreteFilter  Numerator=[0 Ts]  Denominator=[1 -1]  InitialStates=Q0  SampleTime=Ts
  y : Outport
  dy : Outport  Port=2
  wires:
  Discrete FIR Filter1/1 -> Discrete Filter/1, dy/1
  x/1 -> Discrete FIR Filter1/1
  Discrete Filter/1 -> y/1

== system TrajectoryGenerator2DOF/Trajectory Generator/M23 ==
  x : Inport
  Discrete FIR Filter1 : DiscreteFir  Coefficients=1/N/Ts*[1 zeros(1,N-1) -1]  InitialStates=Q0  SampleTime=Ts
  Discrete Filter : DiscreteFilter  Numerator=[0 Ts]  Denominator=[1 -1]  InitialStates=Q0  SampleTime=Ts
  y : Outport
  dy : Outport  Port=2
  wires:
  Discrete FIR Filter1/1 -> Discrete Filter/1, dy/1
  x/1 -> Discrete FIR Filter1/1
  Discrete Filter/1 -> y/1

== system TrajectoryGenerator2DOF/Trajectory Generator/M24 ==
  x : Inport
  Discrete FIR Filter1 : DiscreteFir  Coefficients=1/N/Ts*[1 zeros(1,N-1) -1]  InitialStates=Q0  SampleTime=Ts
  Discrete Filter : DiscreteFilter  Numerator=[0 Ts]  Denominator=[1 -1]  InitialStates=Q0  SampleTime=Ts
  y : Outport
  dy : Outport  Port=2
  wires:
  Discrete FIR Filter1/1 -> Discrete Filter/1, dy/1
  x/1 -> Discrete FIR Filter1/1
  Discrete Filter/1 -> y/1

== system TrajectoryGenerator2DOF/Trajectory Generator/M33 ==
  x : Inport
  Discrete FIR Filter1 : DiscreteFir  Coefficients=1/N/Ts*[1 zeros(1,N-1) -1]  InitialStates=Q0  SampleTime=Ts
  Discrete Filter : DiscreteFilter  Numerator=[0 Ts]  Denominator=[1 -1]  InitialStates=Q0  SampleTime=Ts
  y : Outport
  dy : Outport  Port=2
  wires:
  Discrete FIR Filter1/1 -> Discrete Filter/1, dy/1
  x/1 -> Discrete FIR Filter1/1
  Discrete Filter/1 -> y/1

== system TrajectoryGenerator2DOF/Trajectory Generator/M34 ==
  x : Inport
  Discrete FIR Filter1 : DiscreteFir  Coefficients=1/N/Ts*[1 zeros(1,N-1) -1]  InitialStates=Q0  SampleTime=Ts
  Discrete Filter : DiscreteFilter  Numerator=[0 Ts]  Denominator=[1 -1]  InitialStates=Q0  SampleTime=Ts
  y : Outport
  dy : Outport  Port=2
  wires:
  Discrete FIR Filter1/1 -> Discrete Filter/1, dy/1
  x/1 -> Discrete FIR Filter1/1
  Discrete Filter/1 -> y/1

== system TrajectoryGenerator2DOF/Trajectory Generator/M44 ==
  x : Inport
  Discrete FIR Filter1 : DiscreteFir  Coefficients=1/N/Ts*[1 zeros(1,N-1) -1]  InitialStates=Q0  SampleTime=Ts
  Discrete Filter : DiscreteFilter  Numerator=[0 Ts]  Denominator=[1 -1]  InitialStates=Q0  SampleTime=Ts
  y : Outport
  dy : Outport  Port=2
  wires:
  Discrete FIR Filter1/1 -> Discrete Filter/1, dy/1
  x/1 -> Discrete FIR Filter1/1
  Discrete Filter/1 -> y/1

== system TrajectoryGenerator2DOF/Trajectory Generator1/M11 ==
  x : Inport
  Discrete FIR Filter1 : DiscreteFir  Coefficients=1/N/Ts*[1 zeros(1,N-1) -1]  InitialStates=Q0  SampleTime=Ts
  Discrete Filter : DiscreteFilter  Numerator=[0 Ts]  Denominator=[1 -1]  InitialStates=Q0  SampleTime=Ts
  y : Outport
  dy : Outport  Port=2
  wires:
  Discrete Filter/1 -> y/1
  x/1 -> Discrete FIR Filter1/1
  Discrete FIR Filter1/1 -> dy/1, Discrete Filter/1

== system TrajectoryGenerator2DOF/Trajectory Generator1/M12 ==
  x : Inport
  Discrete FIR Filter1 : DiscreteFir  Coefficients=1/N/Ts*[1 zeros(1,N-1) -1]  InitialStates=Q0  SampleTime=Ts
  Discrete Filter : DiscreteFilter  Numerator=[0 Ts]  Denominator=[1 -1]  InitialStates=Q0  SampleTime=Ts
  y : Outport
  dy : Outport  Port=2
  wires:
  Discrete Filter/1 -> y/1
  x/1 -> Discrete FIR Filter1/1
  Discrete FIR Filter1/1 -> dy/1, Discrete Filter/1

== system TrajectoryGenerator2DOF/Trajectory Generator1/M13 ==
  x : Inport
  Discrete FIR Filter1 : DiscreteFir  Coefficients=1/N/Ts*[1 zeros(1,N-1) -1]  InitialStates=Q0  SampleTime=Ts
  Discrete Filter : DiscreteFilter  Numerator=[0 Ts]  Denominator=[1 -1]  InitialStates=Q0  SampleTime=Ts
  y : Outport
  dy : Outport  Port=2
  wires:
  Discrete Filter/1 -> y/1
  x/1 -> Discrete FIR Filter1/1
  Discrete FIR Filter1/1 -> dy/1, Discrete Filter/1

== system TrajectoryGenerator2DOF/Trajectory Generator1/M14 ==
  x : Inport
  Discrete FIR Filter1 : DiscreteFir  Coefficients=1/N/Ts*[1 zeros(1,N-1) -1]  InitialStates=Q0  SampleTime=Ts
  Discrete Filter : DiscreteFilter  Numerator=[0 Ts]  Denominator=[1 -1]  InitialStates=Q0  SampleTime=Ts
  y : Outport
  dy : Outport  Port=2
  wires:
  Discrete Filter/1 -> y/1
  x/1 -> Discrete FIR Filter1/1
  Discrete FIR Filter1/1 -> dy/1, Discrete Filter/1

== system TrajectoryGenerator2DOF/Trajectory Generator1/M22 ==
  x : Inport
  Discrete FIR Filter1 : DiscreteFir  Coefficients=1/N/Ts*[1 zeros(1,N-1) -1]  InitialStates=Q0  SampleTime=Ts
  Discrete Filter : DiscreteFilter  Numerator=[0 Ts]  Denominator=[1 -1]  InitialStates=Q0  SampleTime=Ts
  y : Outport
  dy : Outport  Port=2
  wires:
  Discrete Filter/1 -> y/1
  x/1 -> Discrete FIR Filter1/1
  Discrete FIR Filter1/1 -> dy/1, Discrete Filter/1

== system TrajectoryGenerator2DOF/Trajectory Generator1/M23 ==
  x : Inport
  Discrete FIR Filter1 : DiscreteFir  Coefficients=1/N/Ts*[1 zeros(1,N-1) -1]  InitialStates=Q0  SampleTime=Ts
  Discrete Filter : DiscreteFilter  Numerator=[0 Ts]  Denominator=[1 -1]  InitialStates=Q0  SampleTime=Ts
  y : Outport
  dy : Outport  Port=2
  wires:
  Discrete Filter/1 -> y/1
  x/1 -> Discrete FIR Filter1/1
  Discrete FIR Filter1/1 -> dy/1, Discrete Filter/1

== system TrajectoryGenerator2DOF/Trajectory Generator1/M24 ==
  x : Inport
  Discrete FIR Filter1 : DiscreteFir  Coefficients=1/N/Ts*[1 zeros(1,N-1) -1]  InitialStates=Q0  SampleTime=Ts
  Discrete Filter : DiscreteFilter  Numerator=[0 Ts]  Denominator=[1 -1]  InitialStates=Q0  SampleTime=Ts
  y : Outport
  dy : Outport  Port=2
  wires:
  Discrete Filter/1 -> y/1
  x/1 -> Discrete FIR Filter1/1
  Discrete FIR Filter1/1 -> dy/1, Discrete Filter/1

== system TrajectoryGenerator2DOF/Trajectory Generator1/M33 ==
  x : Inport
  Discrete FIR Filter1 : DiscreteFir  Coefficients=1/N/Ts*[1 zeros(1,N-1) -1]  InitialStates=Q0  SampleTime=Ts
  Discrete Filter : DiscreteFilter  Numerator=[0 Ts]  Denominator=[1 -1]  InitialStates=Q0  SampleTime=Ts
  y : Outport
  dy : Outport  Port=2
  wires:
  Discrete Filter/1 -> y/1
  x/1 -> Discrete FIR Filter1/1
  Discrete FIR Filter1/1 -> dy/1, Discrete Filter/1

== system TrajectoryGenerator2DOF/Trajectory Generator1/M34 ==
  x : Inport
  Discrete FIR Filter1 : DiscreteFir  Coefficients=1/N/Ts*[1 zeros(1,N-1) -1]  InitialStates=Q0  SampleTime=Ts
  Discrete Filter : DiscreteFilter  Numerator=[0 Ts]  Denominator=[1 -1]  InitialStates=Q0  SampleTime=Ts
  y : Outport
  dy : Outport  Port=2
  wires:
  Discrete Filter/1 -> y/1
  x/1 -> Discrete FIR Filter1/1
  Discrete FIR Filter1/1 -> dy/1, Discrete Filter/1

== system TrajectoryGenerator2DOF/Trajectory Generator1/M44 ==
  x : Inport
  Discrete FIR Filter1 : DiscreteFir  Coefficients=1/N/Ts*[1 zeros(1,N-1) -1]  InitialStates=Q0  SampleTime=Ts
  Discrete Filter : DiscreteFilter  Numerator=[0 Ts]  Denominator=[1 -1]  InitialStates=Q0  SampleTime=Ts
  y : Outport
  dy : Outport  Port=2
  wires:
  Discrete Filter/1 -> y/1
  x/1 -> Discrete FIR Filter1/1
  Discrete FIR Filter1/1 -> dy/1, Discrete Filter/1

== system TrajectoryGenerator2DOF/Trajectory Generator10/M11 ==
  x : Inport
  Discrete FIR Filter1 : DiscreteFir  Coefficients=1/N/Ts*[1 zeros(1,N-1) -1]  InitialStates=Q0  SampleTime=Ts
  Discrete Filter : DiscreteFilter  Numerator=[0 Ts]  Denominator=[1 -1]  InitialStates=Q0  SampleTime=Ts
  y : Outport
  dy : Outport  Port=2
  wires:
  Discrete FIR Filter1/1 -> Discrete Filter/1, dy/1
  x/1 -> Discrete FIR Filter1/1
  Discrete Filter/1 -> y/1

== system TrajectoryGenerator2DOF/Trajectory Generator10/M12 ==
  x : Inport
  Discrete FIR Filter1 : DiscreteFir  Coefficients=1/N/Ts*[1 zeros(1,N-1) -1]  InitialStates=Q0  SampleTime=Ts
  Discrete Filter : DiscreteFilter  Numerator=[0 Ts]  Denominator=[1 -1]  InitialStates=Q0  SampleTime=Ts
  y : Outport
  dy : Outport  Port=2
  wires:
  Discrete FIR Filter1/1 -> Discrete Filter/1, dy/1
  x/1 -> Discrete FIR Filter1/1
  Discrete Filter/1 -> y/1

== system TrajectoryGenerator2DOF/Trajectory Generator10/M13 ==
  x : Inport
  Discrete FIR Filter1 : DiscreteFir  Coefficients=1/N/Ts*[1 zeros(1,N-1) -1]  InitialStates=Q0  SampleTime=Ts
  Discrete Filter : DiscreteFilter  Numerator=[0 Ts]  Denominator=[1 -1]  InitialStates=Q0  SampleTime=Ts
  y : Outport
  dy : Outport  Port=2
  wires:
  Discrete FIR Filter1/1 -> Discrete Filter/1, dy/1
  x/1 -> Discrete FIR Filter1/1
  Discrete Filter/1 -> y/1

== system TrajectoryGenerator2DOF/Trajectory Generator10/M14 ==
  x : Inport
  Discrete FIR Filter1 : DiscreteFir  Coefficients=1/N/Ts*[1 zeros(1,N-1) -1]  InitialStates=Q0  SampleTime=Ts
  Discrete Filter : DiscreteFilter  Numerator=[0 Ts]  Denominator=[1 -1]  InitialStates=Q0  SampleTime=Ts
  y : Outport
  dy : Outport  Port=2
  wires:
  Discrete FIR Filter1/1 -> Discrete Filter/1, dy/1
  x/1 -> Discrete FIR Filter1/1
  Discrete Filter/1 -> y/1

== system TrajectoryGenerator2DOF/Trajectory Generator10/M22 ==
  x : Inport
  Discrete FIR Filter1 : DiscreteFir  Coefficients=1/N/Ts*[1 zeros(1,N-1) -1]  InitialStates=Q0  SampleTime=Ts
  Discrete Filter : DiscreteFilter  Numerator=[0 Ts]  Denominator=[1 -1]  InitialStates=Q0  SampleTime=Ts
  y : Outport
  dy : Outport  Port=2
  wires:
  Discrete FIR Filter1/1 -> Discrete Filter/1, dy/1
  x/1 -> Discrete FIR Filter1/1
  Discrete Filter/1 -> y/1
